simulink model "microgrid_y24f_step10"  (R2024b)
settings: Solver=ode45  StartTime=0.0  StopTime=simu.endTime  MaxStep=simu.maxStepSize  RelTol=1e-3
undefined symbols (not defined in the file or in its folder): es, ht, mg, pv, wp, wt
libraries: simulink x1
settings Model: Creator=tedbrekken  LastModifiedBy=kerrychen
settings RTWCC: GPUComputeCapability=3.5

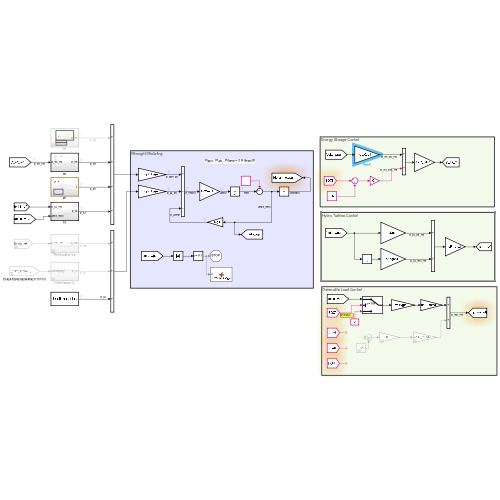
[thumbnail: Simulink's stored preview of the top-level diagram]
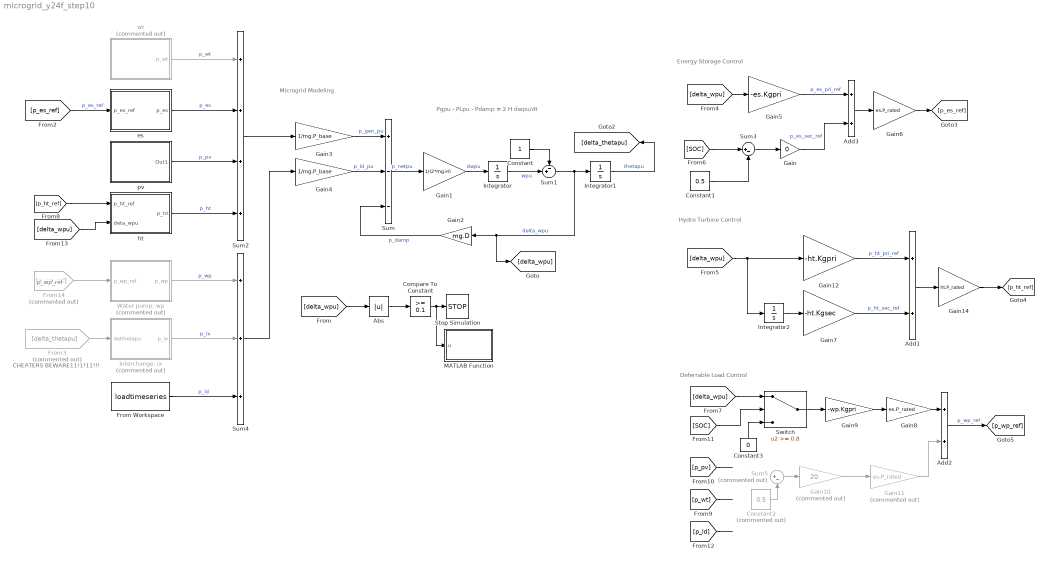
== system microgrid_y24f_step10 ==
  note: p_wp_ref
  note: CHEATERS BEWARE11!1!11!!!
  note: Microgrid Modeling
  note: Pgpu - PLpu - Pdamp = 2 H dwpu/dt
  note: Deferrable Load Control
  note: Hydro Turbine Control
  note: Energy Storage Control
  Abs : Abs  SaturateOnIntegerOverflow=off
  Add1 : Sum
  Add2 : Sum
  Add3 : Sum
  Compare To Constant : simulink/Logic and Bit Operations/Compare To Constant  relop=>=  const=0.1  OutDataTypeStr=boolean
  Constant : Constant
  Constant1 : Constant  Value=0.5
  Constant2 : Constant  Commented=on  Value=0.5
  Constant3 : Constant  Value=0
  From Workspace : FromWorkspace  VariableName=loadtimeseries  OutputAfterFinalValue=Setting to zero
  From14 : From  Commented=on  GotoTag=p_wp_ref
  From3 : From  Commented=on  GotoTag=delta_thetapu
  Gain : Gain  Gain=0
  Gain1 : Gain  Gain=1/(2*mg.H)
  Gain10 : Gain  Commented=on  Gain=20
  Gain11 : Gain  Commented=on  Gain=es.P_rated
  Gain12 : Gain  Gain=-ht.Kgpri
  Gain14 : Gain  Gain=ht.P_rated
  Gain2 : Gain  Gain=mg.D
  Gain3 : Gain  Gain=1/mg.P_base
  Gain4 : Gain  Gain=1/mg.P_base
  Gain5 : Gain  Gain=-es.Kgpri
  Gain6 : Gain  Gain=es.P_rated
  Gain7 : Gain  Gain=-ht.Kgsec
  Gain8 : Gain  Gain=es.P_rated
  Gain9 : Gain  Gain=-wp.Kgpri
  Integrator : Integrator  InitialCondition=mg.wpu_0
  Integrator1 : Integrator  InitialCondition=mg.wpu_0
  Integrator2 : Integrator
  Interchange: ix : Subsystem  Commented=on
  MATLAB Function : MATLAB Function  TreatAsAtomicUnit=on
  Stop Simulation : Stop
  Sum : Sum  Inputs=+--
  Sum1 : Sum  Inputs=-+|
  Sum2 : Sum  Inputs=++++
  Sum3 : Sum  Inputs=|+-
  Sum4 : Sum  Inputs=+++
  Sum5 : Sum  Commented=on  Inputs=|+-
  Switch : Switch  Threshold=0.8  SaturateOnIntegerOverflow=off  InputSameDT=off
  Water pump: wp : Subsystem  Commented=on
  es : Subsystem
  ht : Subsystem
  pv : Subsystem
  wt : Subsystem  Commented=on
  wires:
  Sum/1 -> Gain1/1  "p_netpu"
  Gain1/1 -> Integrator/1  "dwpu"
  Integrator/1 -> Sum1/2  "wpu"
  Constant/1 -> Sum1/1
  Sum1/1 -> Integrator1/1, [delta_wpu], Gain2/1  "delta_wpu"
  Gain2/1 -> Sum/3  "p_damp"
  Gain3/1 -> Sum/1  "p_gen_pu"
  Gain4/1 -> Sum/2  "p_ld_pu"
  wt/1(p_wt) -> Sum2/1  "p_wt"
  es/1(p_es) -> Sum2/2  "p_es"
  Sum2/1 -> Gain3/1
  From Workspace/1 -> Sum4/3  "p_ld"
  [delta_wpu] -> Abs/1
  Abs/1 -> Compare To Constant/1
  Compare To Constant/1 -> MATLAB Function/1(u), Stop Simulation/1
  [p_es_ref] -> es/1(p_es_ref)  "p_es_ref"
  pv/1(Out1) -> Sum2/3  "p_pv"
  ht/1(p_ht) -> Sum2/4  "p_ht"
  Water pump: wp/1(p_wp) -> Sum4/1  "p_wp"
  Interchange: ix/1(p_ix) -> Sum4/2  "p_ix"
  Integrator1/1 -> [delta_thetapu]  "thetapu"
  From3/1 -> Interchange: ix/1(delthetapu)
  Gain7/1 -> Add1/2  "p_ht_sec_ref"
  Gain12/1 -> Add1/1  "p_ht_pri_ref"
  Gain/1 -> Add3/2  "p_es_sec_ref"
  [p_ld] -> ?
  [delta_wpu] -> Integrator2/1, Gain12/1
  [p_pv] -> ?
  Gain5/1 -> Add3/1  "p_es_pri_ref"
  [delta_wpu] -> Gain5/1
  Add3/1 -> Gain6/1
  [p_wt] -> ?
  Add1/1 -> Gain14/1
  Integrator2/1 -> Gain7/1
  Gain6/1 -> [p_es_ref]
  Gain14/1 -> [p_ht_ref]
  [p_ht_ref] -> ht/1(p_ht_ref)
  [delta_wpu] -> ht/2(deta_wpu)
  From14/1 -> Water pump: wp/1(p_wp_ref)
  [SOC] -> Sum3/1
  Constant1/1 -> Sum3/2
  Sum3/1 -> Gain/1
  Sum4/1 -> Gain4/1
  Add2/1 -> [p_wp_ref]  "p_wp_ref"
  [delta_wpu] -> Switch/1
  Gain9/1 -> Gain8/1
  Gain8/1 -> Add2/1
  Gain11/1 -> Add2/2
  Sum5/1 -> Gain10/1
  [SOC] -> Switch/2
  Constant2/1 -> Sum5/2
  Gain10/1 -> Gain11/1
  Switch/1 -> Gain9/1
  Constant3/1 -> Switch/3

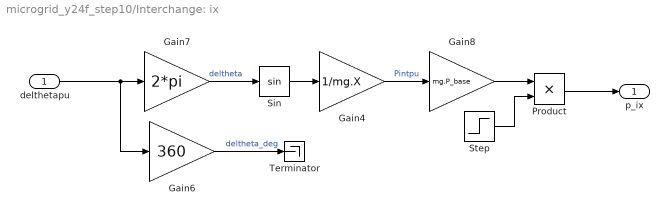
== system microgrid_y24f_step10/Interchange: ix ==
  delthetapu : Inport
  Gain4 : Gain  Gain=1/mg.X
  Gain6 : Gain  Gain=360
  Gain7 : Gain  Gain=2*pi
  Gain8 : Gain  Gain=mg.P_base
  Product : Product
  Sin : Trigonometry
  Step : Step  Time=12*60*60  Before=1  After=0  SampleTime=0
  Terminator : Terminator
  p_ix : Outport
  wires:
  Gain8/1 -> Product/1
  Product/1 -> p_ix/1
  Step/1 -> Product/2
  Gain7/1 -> Sin/1  "deltheta"
  Gain6/1 -> Terminator/1  "deltheta_deg"
  delthetapu/1 -> Gain6/1, Gain7/1
  Sin/1 -> Gain4/1
  Gain4/1 -> Gain8/1  "Pintpu"

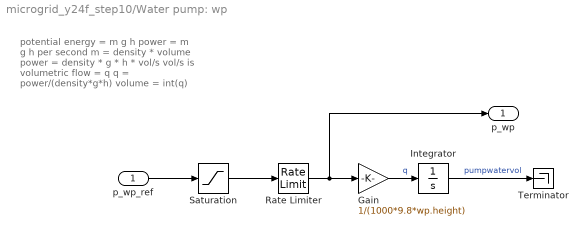
== system microgrid_y24f_step10/Water pump: wp ==
  note: potential energy = m g h
      | power = m g h per second
      | m = density * volume
      |
      | power = density * g * h * vol/s
      |
      | vol/s is volumetric flow = q
      |
      | q = power/(density*g*h)
      |
      | volume = int(q)
  p_wp_ref : Inport
  Gain : Gain  Gain=1/(1000*9.8*wp.height)
  Integrator : Integrator
  Rate Limiter : RateLimiter  RisingSlewLimit=wp.P_upperRate  FallingSlewLimit=wp.P_lowerRate  SampleTimeMode=inherited
  Saturation : Saturate  UpperLimit=wp.P_upper  LowerLimit=wp.P_lower
  Terminator : Terminator
  p_wp : Outport
  wires:
  Rate Limiter/1 -> p_wp/1, Gain/1
  p_wp_ref/1 -> Saturation/1
  Saturation/1 -> Rate Limiter/1
  Gain/1 -> Integrator/1  "q"
  Integrator/1 -> Terminator/1  "pumpwatervol"

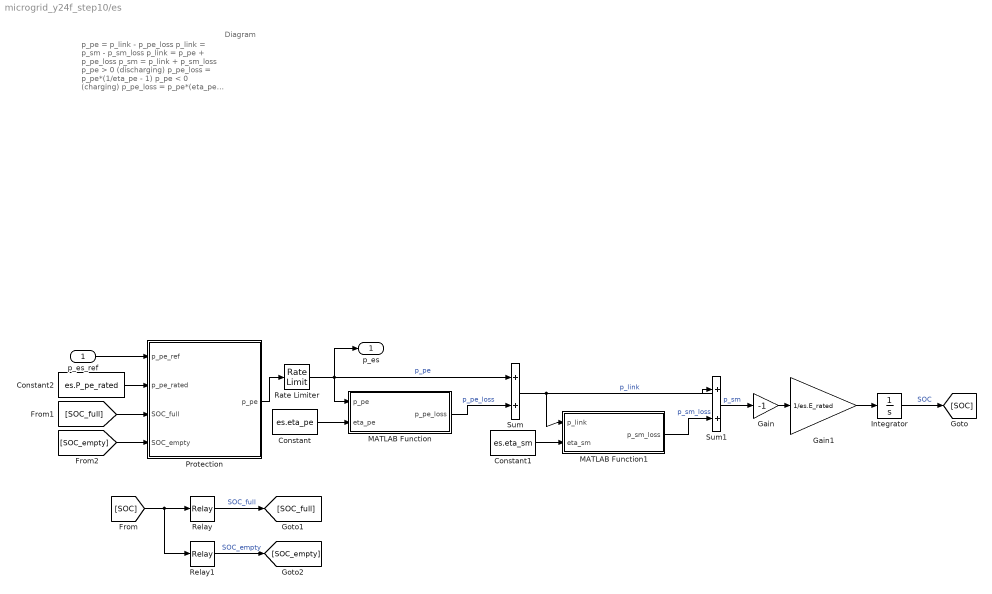
== system microgrid_y24f_step10/es ==
  note: Diagram
  note: p_pe = p_link - p_pe_loss
      | p_link = p_sm - p_sm_loss
      |
      | p_link = p_pe + p_pe_loss
      | p_sm = p_link + p_sm_loss
      |
      | p_pe > 0 (discharging)
      | p_pe_loss = p_pe*(1/eta_pe - 1)
      |
      | p_pe < 0 (charging)
      | p_pe_loss = p_pe*(eta_pe - 1)
      |
      | p_link > 0 (discharging)
      | p_sm_loss = p_link*(1/eta_sm - 1)
      |
      | p_link < 0 (charging)
      | p_sm_loss = p_link*(eta_sm - 1)
      |
      | e_sm = - int(p_sm)
      |
      | SOC = e_sm / es.E_rated
      |
      | if p_pe_ref > p_pe_upper
      | p_pe = p_pe_upper
      |
      | if p_pe_ref < p_pe_lower
      | p_pe = p_pe_lower
      |
      | if SOC >= 1
      | p_pe_lower = 0
      |
      | if SOC <= 0
      | p_pe_upper = 0
  p_es_ref : Inport
  Constant : Constant  Value=es.eta_pe
  Constant1 : Constant  Value=es.eta_sm
  Constant2 : Constant  Value=es.P_pe_rated
  Gain : Gain  Gain=-1
  Gain1 : Gain  Gain=1/es.E_rated
  Integrator : Integrator  InitialCondition=es.SOC_0
  MATLAB Function : MATLAB Function  TreatAsAtomicUnit=on
  MATLAB Function1 : MATLAB Function  TreatAsAtomicUnit=on
  Protection : MATLAB Function  TreatAsAtomicUnit=on
  Rate Limiter : RateLimiter  RisingSlewLimit=es.P_pe_slew_upper  FallingSlewLimit=es.P_pe_slew_lower  SampleTimeMode=inherited
  Relay : Relay  OnSwitchValue=1.01  OffSwitchValue=0.99
  Relay1 : Relay  OnSwitchValue=0.01  OffSwitchValue=-0.01  OnOutputValue=0  OffOutputValue=1
  Sum : Sum
  Sum1 : Sum
  p_es : Outport
  wires:
  [SOC_empty] -> Protection/4(SOC_empty)
  Relay1/1 -> [SOC_empty]  "SOC_empty"
  [SOC_full] -> Protection/3(SOC_full)
  Gain1/1 -> Integrator/1
  Relay/1 -> [SOC_full]  "SOC_full"
  Gain/1 -> Gain1/1
  Constant/1 -> MATLAB Function/2(eta_pe)
  [SOC] -> Relay1/1, Relay/1
  Constant2/1 -> Protection/2(p_pe_rated)
  MATLAB Function/1(p_pe_loss) -> Sum/2  "p_pe_loss"
  Constant1/1 -> MATLAB Function1/2(eta_sm)
  p_es_ref/1 -> Protection/1(p_pe_ref)
  MATLAB Function1/1(p_sm_loss) -> Sum1/2  "p_sm_loss"
  Integrator/1 -> [SOC]  "SOC"
  Sum1/1 -> Gain/1  "p_sm"
  Sum/1 -> MATLAB Function1/1(p_link), Sum1/1  "p_link"
  Protection/1(p_pe) -> Rate Limiter/1
  Rate Limiter/1 -> p_es/1, Sum/1, MATLAB Function/1(p_pe)  "p_pe"

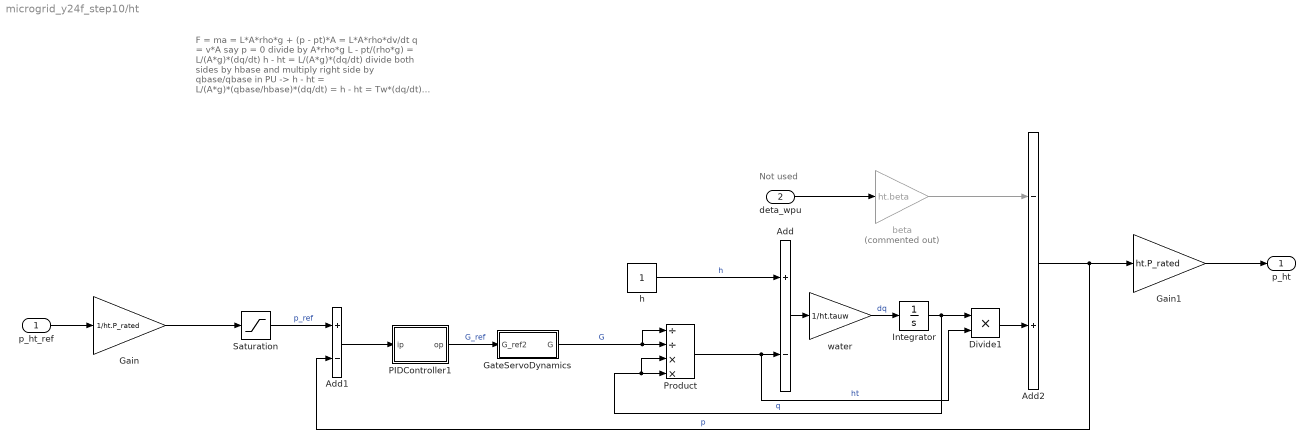
== system microgrid_y24f_step10/ht ==
  note: Not used
  note: F = ma = L*A*rho*g + (p - pt)*A = L*A*rho*dv/dt
      |
      | q = v*A
      |
      | say p = 0
      |
      | divide by A*rho*g
      |
      | L - pt/(rho*g) = L/(A*g)*(dq/dt)
      |
      | h - ht = L/(A*g)*(dq/dt)
      |
      | divide both sides by hbase and multiply right side by qbase/qbase
      |
      | in PU -> h - ht = L/(A*g)*(qbase/hbase)*(dq/dt) = h - ht = Tw*(dq/dt)
      |
      | ht = (q/G)^2
      |
      | pt = ht*q - beta*delta_w
      |
      | Increase in speed changes decreases relative angle of water attack on runner and decreases power
      | and vice versa
  p_ht_ref : Inport
  deta_wpu : Inport  Port=2
  Add : Sum  Inputs=+-
  Add1 : Sum  Inputs=+-
  Add2 : Sum  Inputs=-+
  Divide1 : Product  Inputs=**
  Gain : Gain  Gain=1/ht.P_rated
  Gain1 : Gain  Gain=ht.P_rated
  GateServoDynamics : Subsystem
  Integrator : Integrator  InitialCondition=ht.q_0
  PIDController1 : Subsystem  mask{kp=ht.powercontroller.kp, ki=ht.powercontroller.ki, kd=ht.powercontroller.kd, kt=ht.powercontroller.kt, Td=ht.powercontroller.Td, upperLimit=ht.powercontroller.upperLimit, lowerLimit=ht.powercontroller.lowerLimit, int_0=ht.powercontroller.int_0}
      mask prompts: kp "Proportional gain"; ki "Integral gain"; kd "Derivative gain"; kt "Windup gain"; Td "Derivative time constant"; upperLimit "Upper limit"; lowerLimit "Lower limit"; int_0 "Initial condition"
  Product : Product  Inputs=//**
  Saturation : Saturate  UpperLimit=1  LowerLimit=0
  beta : Gain  Commented=on  Gain=ht.beta
  h : Constant
  water : Gain  Gain=1/ht.tauw
  p_ht : Outport
  wires:
  water/1 -> Integrator/1  "dq"
  deta_wpu/1 -> beta/1
  beta/1 -> Add2/1
  Integrator/1 -> Product/3, Product/4, Divide1/1  "q"
  GateServoDynamics/1(G) -> Product/1, Product/2  "G"
  Product/1 -> Divide1/2, Add/2  "ht"
  Add/1 -> water/1
  h/1 -> Add/1  "h"
  Divide1/1 -> Add2/2
  PIDController1/1(op) -> GateServoDynamics/1(G_ref2)  "G_ref"
  Add2/1 -> Add1/2, Gain1/1  "p"
  Gain1/1 -> p_ht/1
  p_ht_ref/1 -> Gain/1
  Saturation/1 -> Add1/1  "p_ref"
  Gain/1 -> Saturation/1
  Add1/1 -> PIDController1/1(ip)

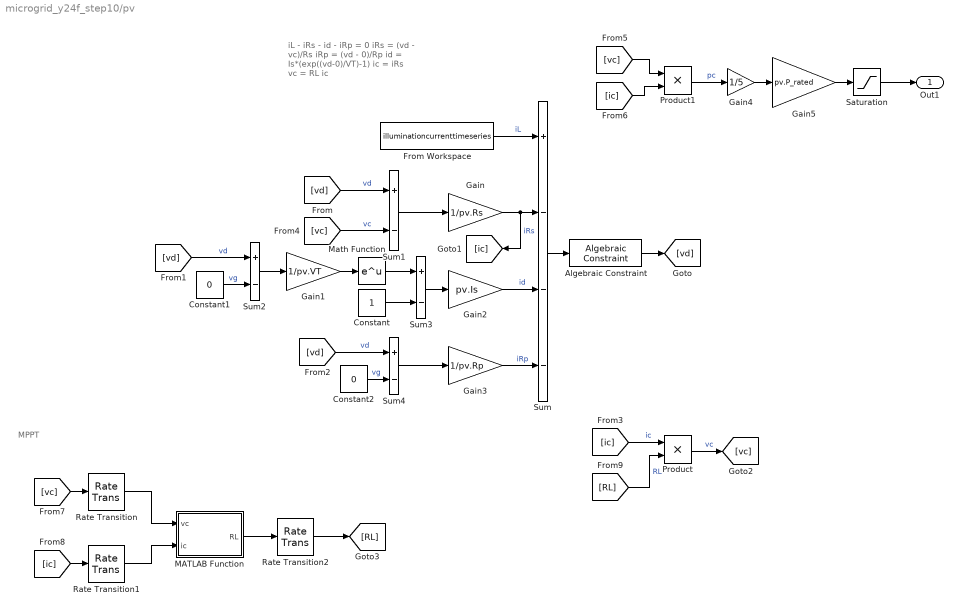
== system microgrid_y24f_step10/pv ==
  note: MPPT
  note: iL - iRs - id - iRp = 0
      |
      | iRs = (vd - vc)/Rs
      |
      | iRp = (vd - 0)/Rp
      |
      | id = Is*(exp((vd-0)/VT)-1)
      |
      | ic = iRs
      |
      | vc = RL ic
  Algebraic Constraint : AlgebraicConstraint  InitialGuess=pv.vd_0
  Constant : Constant
  Constant1 : Constant  Value=0
  Constant2 : Constant  Value=0
  From Workspace : FromWorkspace  VariableName=illuminationcurrenttimeseries  OutputAfterFinalValue=Setting to zero
  Gain : Gain  Gain=1/pv.Rs
  Gain1 : Gain  Gain=1/pv.VT
  Gain2 : Gain  Gain=pv.Is
  Gain3 : Gain  Gain=1/pv.Rp
  Gain4 : Gain  Gain=1/5
  Gain5 : Gain  Gain=pv.P_rated
  MATLAB Function : MATLAB Function  TreatAsAtomicUnit=on
  Math Function : Math
  Product : Product
  Product1 : Product
  Rate Transition : RateTransition  Deterministic=off  OutPortSampleTime=pv.MPPT_sampleTime
  Rate Transition1 : RateTransition  Deterministic=off  OutPortSampleTime=pv.MPPT_sampleTime
  Rate Transition2 : RateTransition  OutPortSampleTime=0
  Saturation : Saturate  UpperLimit=pv.P_rated  LowerLimit=0
  Sum : Sum  Inputs=+---
  Sum{1..4} (4 alike) : Sum  Inputs=+-
  Out1 : Outport
  wires:
  From Workspace/1 -> Sum/1  "iL"
  Gain/1 -> [ic], Sum/2  "iRs"
  Gain2/1 -> Sum/3  "id"
  Sum/1 -> Algebraic Constraint/1
  Sum1/1 -> Gain/1
  [vd] -> Sum1/1  "vd"
  [vc] -> Sum1/2  "vc"
  [vd] -> Sum2/1  "vd"
  Constant1/1 -> Sum2/2  "vg"
  Sum2/1 -> Gain1/1
  Gain1/1 -> Math Function/1
  Math Function/1 -> Sum3/1
  Constant/1 -> Sum3/2
  Sum3/1 -> Gain2/1
  Gain3/1 -> Sum/4  "iRp"
  Constant2/1 -> Sum4/2  "vg"
  Sum4/1 -> Gain3/1
  [vd] -> Sum4/1  "vd"
  Algebraic Constraint/1 -> [vd]
  [ic] -> Product/1  "ic"
  [RL] -> Product/2  "RL"
  Product/1 -> [vc]  "vc"
  [ic] -> Product1/2
  [vc] -> Product1/1
  Product1/1 -> Gain4/1  "pc"
  [vc] -> Rate Transition/1
  [ic] -> Rate Transition1/1
  Rate Transition1/1 -> MATLAB Function/2(ic)
  Rate Transition/1 -> MATLAB Function/1(vc)
  Rate Transition2/1 -> [RL]
  MATLAB Function/1(RL) -> Rate Transition2/1
  Gain5/1 -> Saturation/1
  Saturation/1 -> Out1/1
  Gain4/1 -> Gain5/1

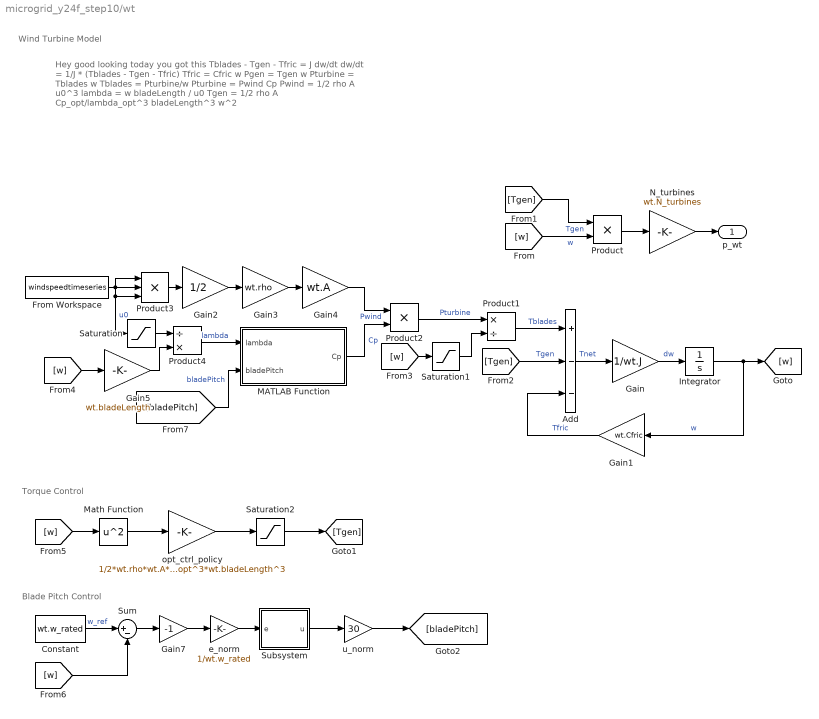
== system microgrid_y24f_step10/wt ==
  note: Blade Pitch Control
  note: Wind Turbine Model
  note: Hey good looking today you got this
      |
      | Tblades - Tgen - Tfric = J dw/dt
      | dw/dt = 1/J * (Tblades - Tgen - Tfric)
      | Tfric = Cfric w
      |
      | Pgen = Tgen w
      |
      | Pturbine = Tblades w
      | Tblades = Pturbine/w
      |
      | Pturbine = Pwind Cp
      |
      | Pwind = 1/2 rho A u0^3
      |
      | lambda = w bladeLength / u0
      |
      | Tgen = 1/2 rho A Cp_opt/lambda_opt^3 bladeLength^3 w^2
  note: Torque Control
  Add : Sum  Inputs=+--
  Constant : Constant  Value=wt.w_rated
  From Workspace : FromWorkspace  VariableName=windspeedtimeseries
  Gain : Gain  Gain=1/wt.J
  Gain1 : Gain  Gain=wt.Cfric
  Gain2 : Gain  Gain=1/2
  Gain3 : Gain  Gain=wt.rho
  Gain4 : Gain  Gain=wt.A
  Gain5 : Gain  Gain=wt.bladeLength
  Gain7 : Gain  Gain=-1
  Integrator : Integrator  InitialCondition=wt.w_0
  MATLAB Function : MATLAB Function  TreatAsAtomicUnit=on
  Math Function : Math  Operator=square
  N_turbines : Gain  Gain=wt.N_turbines
  Product : Product
  Product1 : Product  Inputs=*/
  Product2 : Product
  Product3 : Product  Inputs=3
  Product4 : Product  Inputs=/*
  Saturation : Saturate  UpperLimit=inf  LowerLimit=1e-3
  Saturation1 : Saturate  UpperLimit=inf  LowerLimit=1e-3
  Saturation2 : Saturate  UpperLimit=wt.Tgen_rated  LowerLimit=0
  Subsystem : Subsystem  mask{kp=wt.pitchctrl.kp, ki=wt.pitchctrl.ki, upperLimit=wt.pitchctrl.upperLimit, lowerLimit=wt.pitchctrl.lowerLimit}
      mask prompts: kp "Proportional gain"; ki "Integral gain"; upperLimit "Upper limit"; lowerLimit "Lower limit"
  Sum : Sum  Inputs=|+-
  e_norm : Gain  Gain=1/wt.w_rated
  opt_ctrl_policy : Gain  Gain=1/2*wt.rho*wt.A*wt.Cp_opt/wt.lambda_opt^3*wt.bladeLength^3
  u_norm : Gain  Gain=30
  p_wt : Outport
  wires:
  Constant/1 -> Sum/1  "w_ref"
  Product1/1 -> Add/1  "Tblades"
  Gain2/1 -> Gain3/1
  [w] -> Saturation1/1
  Gain1/1 -> Add/3  "Tfric"
  u_norm/1 -> [bladePitch]
  Sum/1 -> Gain7/1
  Math Function/1 -> opt_ctrl_policy/1
  Product4/1 -> MATLAB Function/1(lambda)  "lambda"
  Saturation/1 -> Product4/1
  [Tgen] -> Product/1  "Tgen"
  Gain4/1 -> Product2/1  "Pwind"
  e_norm/1 -> Subsystem/1(e)
  Add/1 -> Gain/1  "Tnet"
  [w] -> Math Function/1
  MATLAB Function/1(Cp) -> Product2/2  "Cp"
  Saturation1/1 -> Product1/2
  Saturation2/1 -> [Tgen]
  Gain7/1 -> e_norm/1
  [w] -> Sum/2
  opt_ctrl_policy/1 -> Saturation2/1
  Gain5/1 -> Product4/2
  Product/1 -> N_turbines/1
  Subsystem/1(u) -> u_norm/1
  [w] -> Gain5/1
  Product2/1 -> Product1/1  "Pturbine"
  Integrator/1 -> [w], Gain1/1  "w"
  [w] -> Product/2  "w"
  Product3/1 -> Gain2/1
  Gain3/1 -> Gain4/1
  From Workspace/1 -> Saturation/1, Product3/3, Product3/2, Product3/1  "u0"
  [Tgen] -> Add/2  "Tgen"
  [bladePitch] -> MATLAB Function/2(bladePitch)  "bladePitch"
  Gain/1 -> Integrator/1  "dw"
  N_turbines/1 -> p_wt/1

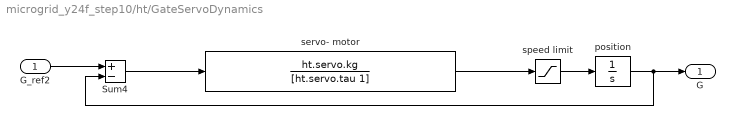
== system microgrid_y24f_step10/ht/GateServoDynamics ==
  G_ref2 : Inport
  Sum4 : Sum  Inputs=+-  InputSameDT=on  SaturateOnIntegerOverflow=on  OutDataTypeStr=Inherit: Same as first input
  position : Integrator  InitialCondition=ht.servo.initPos  LimitOutput=on  UpperSaturationLimit=ht.servo.posUpperLimit  LowerSaturationLimit=ht.servo.posLowerLimit
  servo- motor : TransferFcn  Numerator=ht.servo.kg  Denominator=[ht.servo.tau 1]
  speed limit : Saturate  UpperLimit=ht.servo.speedUpperLimit  LowerLimit=ht.servo.speedLowerLimit
  G : Outport
  wires:
  position/1 -> G/1, Sum4/2
  speed limit/1 -> position/1
  servo- motor/1 -> speed limit/1
  Sum4/1 -> servo- motor/1
  G_ref2/1 -> Sum4/1

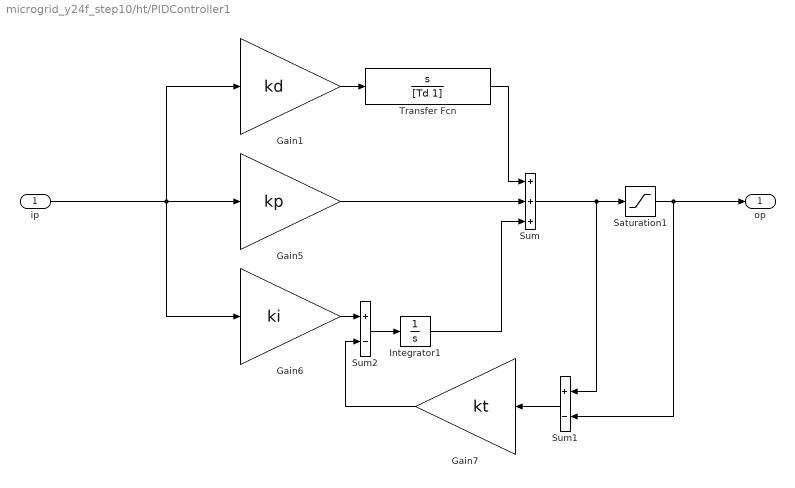
== system microgrid_y24f_step10/ht/PIDController1 ==
  ip : Inport
  Gain1 : Gain  Gain=kd
  Gain5 : Gain  Gain=kp
  Gain6 : Gain  Gain=ki
  Gain7 : Gain  Gain=kt
  Integrator1 : Integrator  InitialCondition=int_0
  Saturation1 : Saturate  UpperLimit=upperLimit  LowerLimit=lowerLimit
  Sum : Sum  Inputs=+++
  Sum1 : Sum  Inputs=+-
  Sum2 : Sum  Inputs=+-
  Transfer Fcn : TransferFcn  Numerator=[1 0]  Denominator=[Td 1]
  op : Outport
  wires:
  Sum2/1 -> Integrator1/1
  Integrator1/1 -> Sum/3
  Gain7/1 -> Sum2/2
  Sum1/1 -> Gain7/1
  Gain6/1 -> Sum2/1
  ip/1 -> Gain1/1, Gain6/1, Gain5/1
  Saturation1/1 -> op/1, Sum1/2
  Gain5/1 -> Sum/2
  Sum/1 -> Sum1/1, Saturation1/1
  Gain1/1 -> Transfer Fcn/1
  Transfer Fcn/1 -> Sum/1

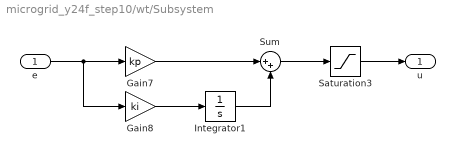
== system microgrid_y24f_step10/wt/Subsystem ==
  e : Inport
  Gain7 : Gain  Gain=kp
  Gain8 : Gain  Gain=ki
  Integrator1 : Integrator  LimitOutput=on  UpperSaturationLimit=upperLimit  LowerSaturationLimit=lowerLimit
  Saturation3 : Saturate  UpperLimit=upperLimit  LowerLimit=lowerLimit
  Sum : Sum  Inputs=|++
  u : Outport
  wires:
  Integrator1/1 -> Sum/2
  Saturation3/1 -> u/1
  e/1 -> Gain8/1, Gain7/1
  Gain8/1 -> Integrator1/1
  Gain7/1 -> Sum/1
  Sum/1 -> Saturation3/1

== matlab function microgrid_y24f_step10/es/MATLAB Function ==
  data: p_pe input; p_pe_loss output; eta_pe input
function p_pe_loss = fcn(p_pe,eta_pe)
% p_pe > 0 (discharging)
% p_pe_loss = p_pe*(1/eta_pe - 1)
%
% p_pe < 0 (charging)
% p_pe_loss = p_pe*(eta_pe - 1)

if p_pe > 0
    p_pe_loss = p_pe*(1/eta_pe-1);
elseif p_pe < 0
    p_pe_loss = p_pe*(eta_pe-1);
elseif p_pe == 0
    p_pe_loss = 0;
else
    error("I didnt think of this")
end

== matlab function microgrid_y24f_step10/wt/MATLAB Function ==
  data: lambda input; Cp output; bladePitch input
function Cp = fcn(lambda,bladePitch)

% https://www.mathworks.com/help/physmod/sps/powersys/ref/windturbine.html

c = [...
    0.5176 ...
    116 ...
    0.4 ...
    5 ...
    21 ...
    0.0068];

if (lambda+0.08*bladePitch) == 0
    lambda = 1e-3;
end

lambdaai = 1/( 1/(lambda+0.08*bladePitch) - 0.035/(bladePitch^3+1) );

Cp = c(1)*(c(2)/lambdaai-c(3)*bladePitch-c(4))*exp(-c(5)/lambdaai) + c(6)*lambda;

== matlab function microgrid_y24f_step10/es/MATLAB Function1 ==
  data: p_link input; p_sm_loss output; eta_sm input
function p_sm_loss = fcn(p_link,eta_sm)
% p_link > 0 (discharging)
% p_sm_loss = p_link*(1/eta_sm - 1)
%
% p_link < 0 (charging)
% p_sm_loss = p_link*(eta_sm - 1)

if p_link > 0
    p_sm_loss = p_link*(1/eta_sm-1);
elseif p_link < 0
    p_sm_loss = p_link*(eta_sm-1);
elseif p_link == 0
    p_sm_loss = 0;
else
    error("I didnt think of this")
end

== matlab function microgrid_y24f_step10/es/Protection ==
  data: p_pe_ref input; p_pe output; p_pe_rated input; SOC_full input; SOC_empty input
function p_pe = fcn(p_pe_ref,p_pe_rated,SOC_full,SOC_empty)
% p_pe_upper = p_pe_rated
% p_pe_lower = -p_pe_rated
%
% if SOC >= 1
% p_pe_lower = 0
% 
% if SOC <= 0
% p_pe_upper = 0
%
% if p_pe_ref > p_pe_upper
% p_pe = p_pe_upper
% 
% if p_pe_ref < p_pe_lower
% p_pe = p_pe_lower

p_pe_upper = p_pe_rated; % 10
p_pe_lower = -p_pe_rated; % -10

if SOC_full
    p_pe_lower = 0; % 0
end

if SOC_empty
    p_pe_upper = 0;
end

if p_pe_ref > p_pe_upper
    p_pe = p_pe_upper;
elseif p_pe_ref < p_pe_lower
    p_pe = p_pe_lower;
else
    p_pe = p_pe_ref;
end

== matlab function microgrid_y24f_step10/MATLAB Function ==
  data: u input
function errormessage(u)

if u == 1
    error("!!!Microgrid exploded due to mismanagement!!!")
end

== matlab function microgrid_y24f_step10/pv/MATLAB Function ==
  data: vc input; RL output; ic input
function RL = mppt(vc,ic)

RLstep = 0.005;

persistent vcprev icprev RLprev directionprev
if isempty(vcprev)
    vcprev = 0;
end
if isempty(icprev)
    icprev = 0;
end
if isempty(RLprev)
    RLprev = 0;
end
if isempty(directionprev)
    directionprev = 1;
end

pc = vc*ic;
pcprev = vcprev*icprev;

% direction -1, 1
if pc > pcprev
    direction = directionprev;
elseif pc < pcprev
    direction = -1*directionprev;
else
    direction = 1;
end

RL = RLprev + direction*RLstep;

% Saturation of control
if RL < 0
    RL = 0;
end
if RL > 5
    RL = 5;
end

% State update
vcprev = vc;
icprev = ic;
directionprev = direction;
RLprev = RL;
